simulink model "AVR_H_inf__"  (R2022a)
settings: Solver=VariableStepAuto  StartTime=0.0  StopTime=150  RelTol=1e-3
libraries: simulink x1
settings Model: Creator=asus  LastModifiedBy=asus

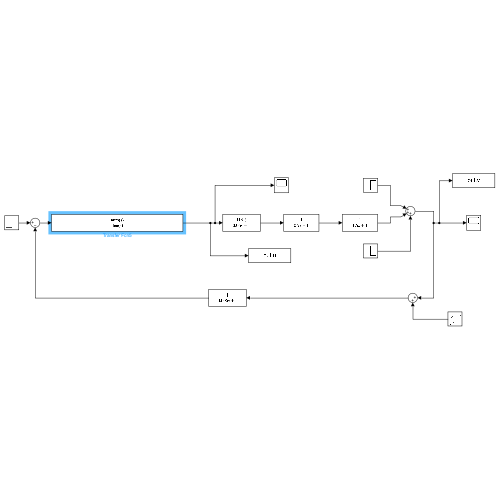
[thumbnail: Simulink's stored preview of the top-level diagram]
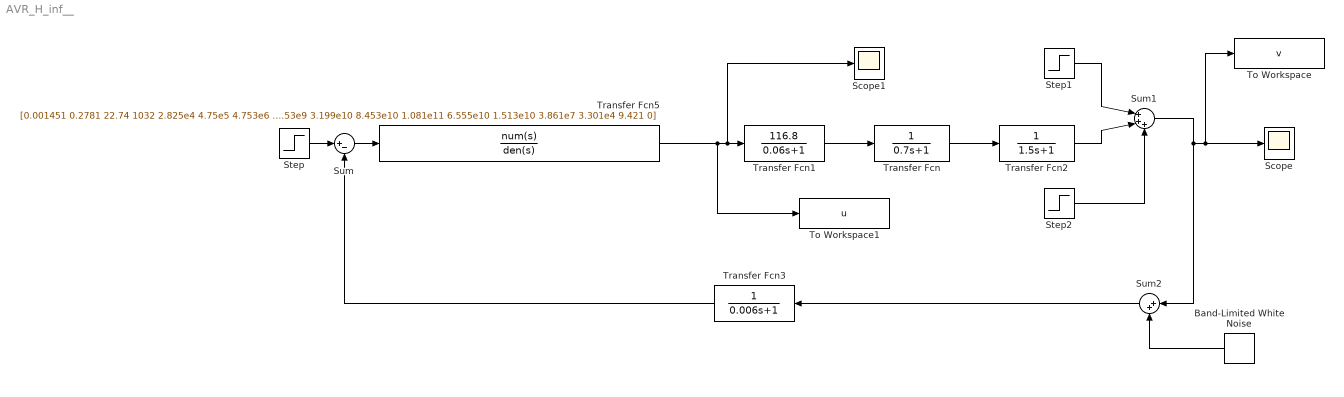
== system AVR_H_inf__ ==
  Band-Limited White Noise : simulink/Sources/Band-Limited White Noise  Cov=[0]  Ts=0.1  seed=[23341]
  Scope : Scope
  Scope1 : Scope
  Step : Step  Time=0  SampleTime=0
  Step1 : Step  Time=50  SampleTime=0
  Step2 : Step  Time=100  After=-1  SampleTime=0
  Sum : Sum  Inputs=|+-
  Sum1 : Sum  Inputs=|+++
  Sum2 : Sum  Inputs=|++
  To Workspace : ToWorkspace  VariableName=v  SaveFormat=Timeseries  SampleTime=-1
  To Workspace1 : ToWorkspace  VariableName=u  SaveFormat=Timeseries  SampleTime=-1
  Transfer Fcn : TransferFcn  Denominator=[0.7 1]
  Transfer Fcn1 : TransferFcn  Numerator=[116.8]  Denominator=[0.06 1]
  Transfer Fcn2 : TransferFcn  Denominator=[1.5 1]
  Transfer Fcn3 : TransferFcn  Denominator=[0.006 1]
  Transfer Fcn5 : TransferFcn  Numerator=[0.001451 0.2781 22.74 1032 2.825e4 4.75e5 4.753e6 2.593e7 6.564e7 8.006e7 4.569e7 9.824e6 2.506e4 21.42 0.006113]  Denominator=[1 212.3 1.913e4 9.507e5 2.835e7 5.154e8 5.53e9 3.199e10 8.453e10 1.081e11 6.555e10 1.513e10 3.861e7 3.301e4 9.421 0]
  wires:
  Transfer Fcn5/1 -> To Workspace1/1, Scope1/1, Transfer Fcn1/1
  Sum/1 -> Transfer Fcn5/1
  Transfer Fcn3/1 -> Sum/2
  Transfer Fcn2/1 -> Sum1/2
  Sum1/1 -> Sum2/1, To Workspace/1, Scope/1
  Step2/1 -> Sum1/3
  Transfer Fcn1/1 -> Transfer Fcn/1
  Step1/1 -> Sum1/1
  Step/1 -> Sum/1
  Transfer Fcn/1 -> Transfer Fcn2/1
  Band-Limited White Noise/1 -> Sum2/2
  Sum2/1 -> Transfer Fcn3/1
